simulink subsystem "tehrani_lung_compartment_v1"  (R2019b)
settings: Solver=VariableStepAuto  StartTime=0.0  StopTime=10.0  RelTol=1e-3
undefined symbols (not defined in the file): __PRM__SERIALIZED__DATA__, C_a_CO2_0, C_a_O2_0, SubsystemReferenceBlock
settings Model: Creator=RH  LastModifiedBy=RH

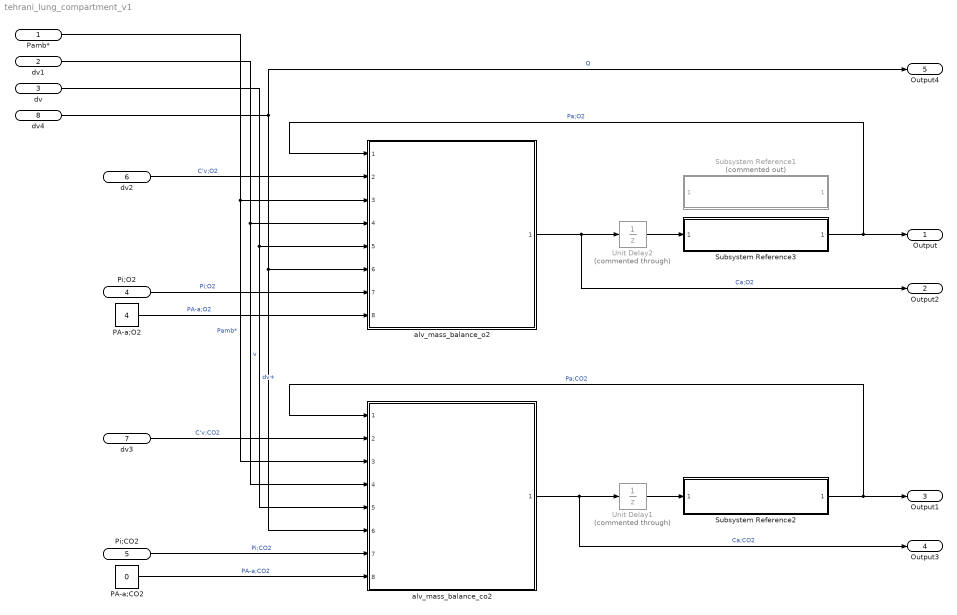
== system tehrani_lung_compartment_v1 ==
  Pamb* : Inport  Unit=mmHg
  dv1 : Inport  Port=2  Unit=L
  dv : Inport  Port=3  Unit=L/s
  Pi;O2 : Inport  Port=4  Unit=mmHg
  Pi;CO2 : Inport  Port=5  Unit=mmHg
  dv2 : Inport  Port=6  Unit=1
  dv3 : Inport  Port=7  Unit=1
  dv4 : Inport  Port=8  Unit=liter/minute
  PA-a;CO2 : Constant  Value=0
  PA-a;O2 : Constant  Value=4
  Subsystem Reference1 : Subsystem  Commented=on  BlockKeywords=__PRM__SERIALIZED__DATA__:SubsystemReferenceBlock  ReferencedSubsystem=O2_dissociation_inv
  Subsystem Reference2 : Subsystem  BlockKeywords=__PRM__SERIALIZED__DATA__:SubsystemReferenceBlock  ReferencedSubsystem=CO2_dissociation_inv
  Subsystem Reference3 : Subsystem  BlockKeywords=__PRM__SERIALIZED__DATA__:SubsystemReferenceBlock  ReferencedSubsystem=O2_dissociation_inv_poly
  Unit Delay1 : UnitDelay  Commented=through  InitialCondition=C_a_CO2_0  SampleTime=-1  HasFrameUpgradeWarning=on
  Unit Delay2 : UnitDelay  Commented=through  InitialCondition=C_a_O2_0  SampleTime=-1  HasFrameUpgradeWarning=on
  alv_mass_balance_co2 : Subsystem  ReferencedSubsystem=tehrani_alv_mass_balance_v3
  alv_mass_balance_o2 : Subsystem  ReferencedSubsystem=tehrani_alv_mass_balance_v3
  Output : Outport  Unit=mmHg
  Output2 : Outport  Port=2  Unit=1
  Output1 : Outport  Port=3  Unit=mmHg
  Output3 : Outport  Port=4  Unit=1
  Output4 : Outport  Port=5  Unit=liter/minute
  wires:
  dv/1 -> alv_mass_balance_o2/5, alv_mass_balance_co2/5  "dv+"
  dv4/1 -> Output4/1, alv_mass_balance_o2/6, alv_mass_balance_co2/6  "Q"
  PA-a;O2/1 -> alv_mass_balance_o2/8  "PA-a;O2"
  Subsystem Reference2/1 -> Output1/1, alv_mass_balance_co2/1  "Pa;CO2"
  alv_mass_balance_o2/1 -> Output2/1, Unit Delay2/1  "Ca;O2"
  dv3/1 -> alv_mass_balance_co2/2  "C'v;CO2"
  Pamb*/1 -> alv_mass_balance_o2/3, alv_mass_balance_co2/3  "Pamb*"
  PA-a;CO2/1 -> alv_mass_balance_co2/8  "PA-a;CO2"
  Pi;CO2/1 -> alv_mass_balance_co2/7  "Pi;CO2"
  Pi;O2/1 -> alv_mass_balance_o2/7  "Pi;O2"
  dv1/1 -> alv_mass_balance_o2/4, alv_mass_balance_co2/4  "v"
  Subsystem Reference3/1 -> Output/1, alv_mass_balance_o2/1  "Pa;O2"
  dv2/1 -> alv_mass_balance_o2/2  "C'v;O2"
  alv_mass_balance_co2/1 -> Unit Delay1/1, Output3/1  "Ca;CO2"
  Unit Delay1/1 -> Subsystem Reference2/1
  Unit Delay2/1 -> Subsystem Reference3/1
